simulink model "MSAP"  (R2023b)
settings: Solver=VariableStepAuto  StartTime=0.0  StopTime=10.0  RelTol=1e-3
undefined symbols (not defined in the file): A1, A2, B1, B2, F, Fie, J, Ld, Lq, P
settings Model: Creator=lylia  LastModifiedBy=lylia

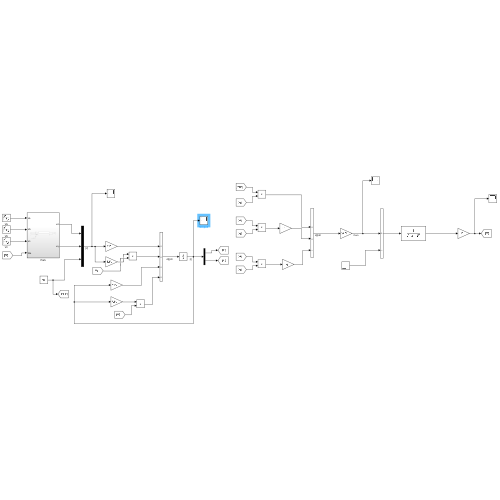
[thumbnail: Simulink's stored preview of the top-level diagram]
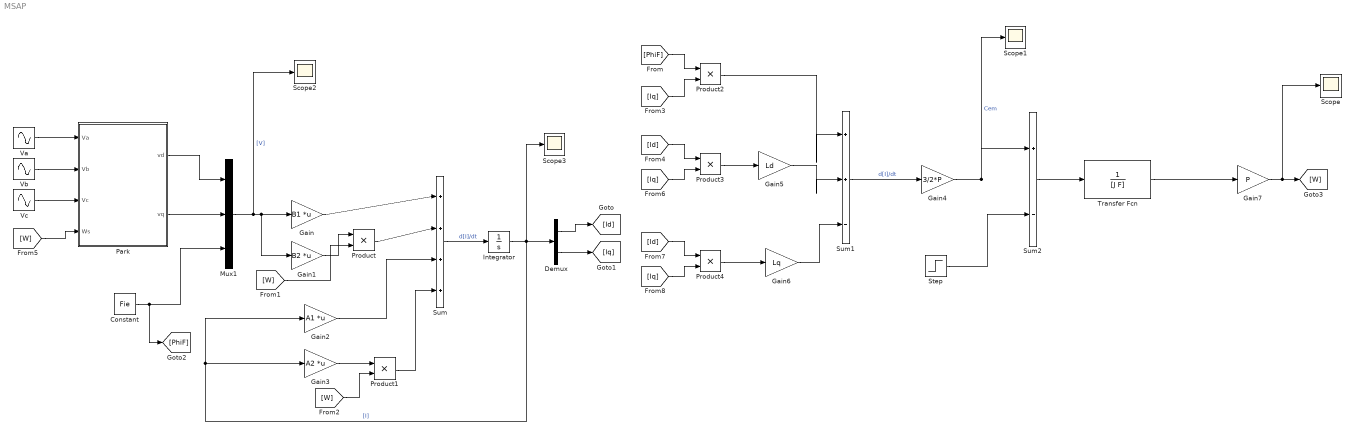
== system MSAP ==
  Constant : Constant  Value=Fie
  Demux : Demux  Outputs=2
  Gain : Gain  Gain=B1  Multiplication=Matrix(K*u)
  Gain1 : Gain  Gain=B2  Multiplication=Matrix(K*u)
  Gain2 : Gain  Gain=A1  Multiplication=Matrix(K*u)
  Gain3 : Gain  Gain=A2  Multiplication=Matrix(K*u)
  Gain4 : Gain  Gain=3/2*P
  Gain5 : Gain  Gain=Ld
  Gain6 : Gain  Gain=Lq
  Gain7 : Gain  Gain=P
  Integrator : Integrator
  Mux1 : Mux  Inputs=3
  Park : Subsystem
  Product{,1..4} (5 alike) : Product
  Scope{,1..3} (4 alike) : Scope
  Step : Step  Time=2  Before=0.5  After=5  SampleTime=0
  Sum : Sum  Inputs=|++++
  Sum1 : Sum  Inputs=|++-
  Sum2 : Sum  Inputs=|+-
  Transfer Fcn : TransferFcn  Denominator=[J F]
  Va : Sin  Amplitude=220*sqrt(2)  Frequency=2*pi*50  SampleTime=0
  Vb : Sin  Amplitude=220*sqrt(2)  Frequency=2*pi*50  Phase=-2*pi/3  SampleTime=0
  Vc : Sin  Amplitude=220*sqrt(2)  Frequency=2*pi*50  Phase=2*pi/3  SampleTime=0
  wires:
  Vb/1 -> Park/2(Vb)
  Vc/1 -> Park/3(Vc)
  Park/1(vd) -> Mux1/1
  Park/2(vq) -> Mux1/2
  [W] -> Park/4(Ws)
  Va/1 -> Park/1(Va)
  Constant/1 -> [PhiF], Mux1/3
  Mux1/1 -> Scope2/1, Gain1/1, Gain/1  "[V]"
  Gain/1 -> Sum/1
  Product/1 -> Sum/2
  Gain1/1 -> Product/1
  [W] -> Product/2
  Gain2/1 -> Sum/3
  Product1/1 -> Sum/4
  Gain3/1 -> Product1/1
  [W] -> Product1/2
  Sum/1 -> Integrator/1  "d[I]/dt"
  Integrator/1 -> Gain3/1, Gain2/1, Scope3/1, Demux/1  "[I]"
  Demux/2 -> [Iq]
  Demux/1 -> [Id]
  [PhiF] -> Product2/1
  [Iq] -> Product2/2
  [Iq] -> Product3/2
  [Id] -> Product3/1
  Product3/1 -> Gain5/1
  [Id] -> Product4/1
  [Iq] -> Product4/2
  Product4/1 -> Gain6/1
  Product2/1 -> Sum1/1
  Gain5/1 -> Sum1/2
  Gain6/1 -> Sum1/3
  Sum1/1 -> Gain4/1  "d[I]/dt"
  Gain4/1 -> Scope1/1, Sum2/1  "Cem"
  Sum2/1 -> Transfer Fcn/1
  Step/1 -> Sum2/2
  Transfer Fcn/1 -> Gain7/1
  Gain7/1 -> Scope/1, [W]

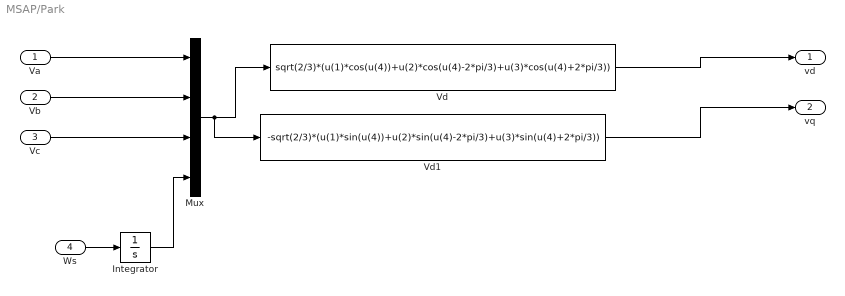
== system MSAP/Park ==
  Va : Inport
  Vb : Inport  Port=2
  Vc : Inport  Port=3
  Ws : Inport  Port=4
  Integrator : Integrator
  Mux : Mux
  Vd : Fcn  Expr=sqrt(2/3)*(u(1)*cos(u(4))+u(2)*cos(u(4)-2*pi/3)+u(3)*cos(u(4)+2*pi/3))
  Vd1 : Fcn  Expr=-sqrt(2/3)*(u(1)*sin(u(4))+u(2)*sin(u(4)-2*pi/3)+u(3)*sin(u(4)+2*pi/3))
  vd : Outport
  vq : Outport  Port=2
  wires:
  Vc/1 -> Mux/3
  Integrator/1 -> Mux/4
  Vb/1 -> Mux/2
  Vd/1 -> vd/1
  Mux/1 -> Vd1/1, Vd/1
  Va/1 -> Mux/1
  Ws/1 -> Integrator/1
  Vd1/1 -> vq/1
